simulink model "FPGA_Comm_control_final"  (Simulink 7.6)
settings: Solver=ode4  StartTime=0.0  StopTime=50  FixedStep=0.01  MaxStep=1e-1  RelTol=1e-3
libraries: simulink x2
settings Model: Creator=jordan  LastModifiedBy=jordan
settings GRTTargetCC: ExtMode=on

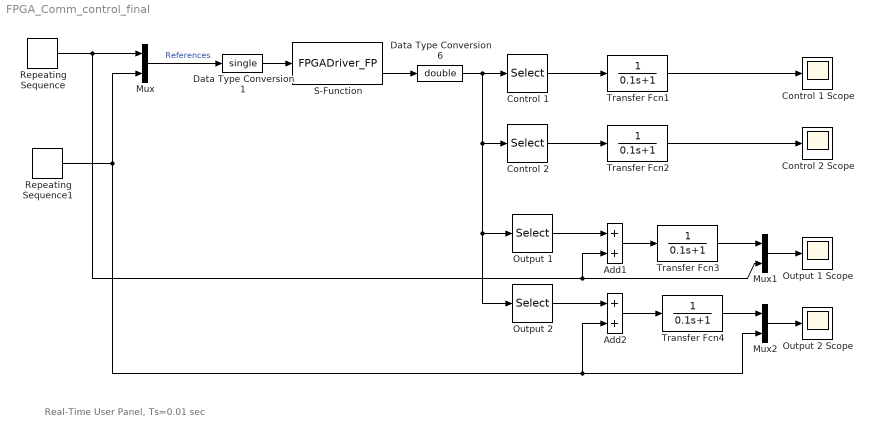
== system FPGA_Comm_control_final ==
  note: Real-Time User Panel, Ts=0.01 sec
  Add1 : Sum
  Add2 : Sum
  Control 1 : Selector  InputPortWidth=4  IndexOptions=Index vector (dialog)  Indices=1  OutputSizes=1
  Control 1 Scope : Scope
      settings: TimeRange=50  YMin=-0.7  YMax=0.8  SaveName=u1  MaxDataPoints=50000
  Control 2 : Selector  InputPortWidth=4  IndexOptions=Index vector (dialog)  Indices=2  OutputSizes=1
  Control 2 Scope : Scope
      settings: TimeRange=50  YMin=-1.5  YMax=1.5  SaveName=u2  MaxDataPoints=50000
  Data Type Conversion1 : DataTypeConversion  OutDataTypeStr=single
  Data Type Conversion6 : DataTypeConversion  OutDataTypeStr=double
  Mux : Mux  Inputs=2
  Mux1 : Mux  Inputs=2
  Mux2 : Mux  Inputs=2
  Output 1 : Selector  InputPortWidth=4  IndexOptions=Index vector (dialog)  Indices=3  OutputSizes=1
  Output 1 Scope : Scope
      settings: TimeRange=50  YMin=-1.5  SaveName=y1  MaxDataPoints=50000
  Output 2 : Selector  InputPortWidth=4  IndexOptions=Index vector (dialog)  Indices=4  OutputSizes=1
  Output 2 Scope : Scope
      settings: TimeRange=50  YMin=-1.5  YMax=5.5  SaveName=y2  MaxDataPoints=50000
  Repeating Sequence : simulink/Sources/Repeating Sequence  SystemSampleTime=-1  rep_seq_t=[0 10 10.1 20 20.1 30 30.1 40]  rep_seq_y=[1 1 0 0 -1 -1 0 0]
  Repeating Sequence1 : simulink/Sources/Repeating Sequence  SystemSampleTime=-1  rep_seq_t=[0 10 10.1 20 20.1 30 30.1 40]  rep_seq_y=[1 1 0 0 -1 -1 0 0]
  S-Function : S-Function  FunctionName=FPGADriver_FP  EnableBusSupport=off
  Transfer Fcn{1..4} (4 alike) : TransferFcn  Denominator=[0.1 1]
  wires:
  S-Function/2 -> Data Type Conversion6/1
  Data Type Conversion1/1 -> S-Function/1
  Data Type Conversion6/1 -> Control 1/1, Control 2/1, Output 1/1, Output 2/1
  Mux/1 -> Data Type Conversion1/1  "References"
  Control 1/1 -> Transfer Fcn1/1
  Control 2/1 -> Transfer Fcn2/1
  Output 1/1 -> Add1/1
  Output 2/1 -> Add2/1
  Repeating Sequence/1 -> Mux/1, Mux1/2, Add1/2
  Mux1/1 -> Output 1 Scope/1
  Mux2/1 -> Output 2 Scope/1
  Add1/1 -> Transfer Fcn3/1
  Add2/1 -> Transfer Fcn4/1
  Repeating Sequence1/1 -> Mux/2, Mux2/2, Add2/2
  Transfer Fcn1/1 -> Control 1 Scope/1
  Transfer Fcn2/1 -> Control 2 Scope/1
  Transfer Fcn3/1 -> Mux1/1
  Transfer Fcn4/1 -> Mux2/1
